simulink model "serratura"  (Simulink 7.2)
settings: Solver=FixedStepDiscrete  StartTime=0.0  StopTime=3  FixedStep=1  RelTol=1e-3  AbsTol=1e-6
settings Model: Creator=prof. G. Celentano  LastModifiedBy=prof. G. Celentano  ExtModeTrigMode=oneshot  ExtModeArmWhenConnect=off
settings DataIOCC: LimitDataPoints=off  SignalLoggingName=sigsOut
settings OptimizationCC: BooleanDataType=off  InitFltsAndDblsToZero=on
settings DebuggingCC: SaveWithParameterizedLinksMsg=none  SignalResolutionControl=TryResolveAllWithWarning  SolverPrmCheckMsg=none  MultiTaskDSMMsg=warning  MultiTaskCondExecSysMsg=none  StrictBusMsg=None
settings HardwareCC: TargetUnknown=on
settings RTWCC: IncludeERTFirstTime=on
settings GRTTargetCC: TargetFcnLib=ansi_tfl_tmw.mat

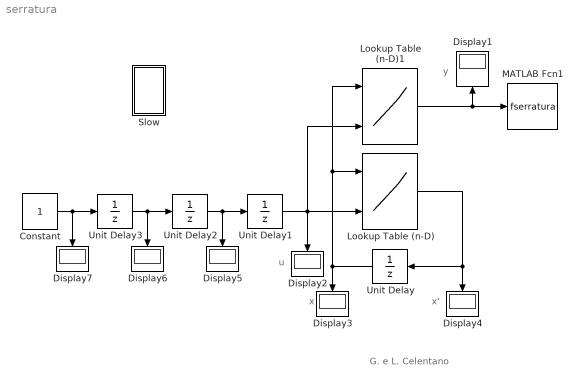
== system serratura ==
  note: G. e L. Celentano
  note: u
  note: x
  note: y
  note: x'
  Constant : Constant  OutDataType=sfix(16)  OutScaling=2^0
  Display{1..7} (7 alike) : Display
      Display1 settings: Orientation=up
      Display2 settings: Orientation=down
      Display3 settings: Orientation=down
      Display4 settings: Orientation=down
      Display5 settings: Orientation=down
      Display6 settings: Orientation=down
      Display7 settings: Orientation=down
  Lookup Table (n-D) : Lookup_n-D  BreakpointsForDimension1=[1 2 3 4]  BreakpointsForDimension2=[1 2 3 4]  IndexSearchMethod=Linear search  Table=[1 1 2 1;1 1 1 3;1 1 4 1;1 1 1 1]  InputSameDT=on
  Lookup Table (n-D)1 : Lookup_n-D  BreakpointsForDimension1=[1 2 3 4]  BreakpointsForDimension2=[1 2 3 4]  IndexSearchMethod=Linear search  Table=[1 1 1 1;1 1 1 1;1 1 1 1;2 1 1 1]  InputSameDT=on
  MATLAB Fcn1 : MATLABFcn  MATLABFcn=fserratura  OutputDimensions=0
  Slow : Subsystem
      mask Display: plot([0 1],[0 1])
  Unit Delay : UnitDelay  Orientation=left  X0=1
  Unit Delay1 : UnitDelay  X0=3
  Unit Delay2 : UnitDelay  X0=4
  Unit Delay3 : UnitDelay  X0=3
  wires:
  Lookup Table (n-D)/1 -> Unit Delay/1, Display4/1
  Unit Delay1/1 -> Lookup Table (n-D)1/2, Display2/1, Lookup Table (n-D)/2
  Lookup Table (n-D)1/1 -> Display1/1, MATLAB Fcn1/1
  Unit Delay2/1 -> Unit Delay1/1, Display5/1
  Unit Delay3/1 -> Unit Delay2/1, Display6/1
  Constant/1 -> Unit Delay3/1, Display7/1
  Unit Delay/1 -> Lookup Table (n-D)1/1, Lookup Table (n-D)/1, Display3/1

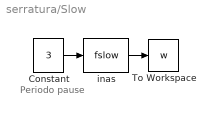
== system serratura/Slow ==
  note: Periodo
      | pause
  Constant : Constant  Value=3  OutDataType=sfix(16)  OutScaling=2^0
  To Workspace : ToWorkspace  VariableName=w  SampleTime=-1  SaveFormat=Array
  inas : MATLABFcn  MATLABFcn=fslow
  wires:
  Constant/1 -> inas/1
  inas/1 -> To Workspace/1
